simulink model "PendulumCart_sim"  (R2015a)
settings: Solver=ode45  StartTime=0.0  StopTime=30.0  RelTol=1e-3
InitFcn:
  | Ts = 0.02;
  | %SMC Parameters
  | lambda = 1; %surface
  | beta = 25;  %pull magnitude
  | U = 0.01;     %saturation
  | %system parameters
  | m = 0.2;
  | M = 0.5;
  | g = 9.8;
  | L = 0.3;
  | %system parameter estimates
  | m_hat = m;
  | M_hat = M;
  | g_hat = g;
  | L_hat = L;
libraries: simulink x1
settings Model: Creator=Logan  LastModifiedBy=Logan

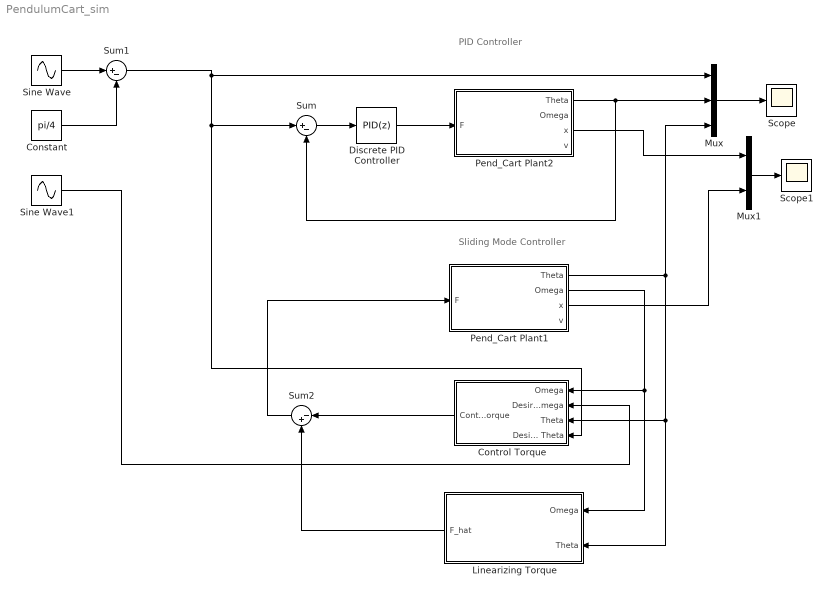
== system PendulumCart_sim ==
  note: PID Controller
  note: Sliding Mode Controller
  Constant : Constant  Value=pi/4
  Control Torque : Subsystem
  Discrete PID Controller : simulink/Continuous/PID Controller  Controller=PID  TimeDomain=Discrete-time  SampleTime=0.01  IntegratorMethod=Forward Euler  FilterMethod=Forward Euler  Form=Parallel  UseFilter=off  ControllerParametersSource=internal  P=100  I=1  D=20  N=250  InitialConditionSource=internal  InitialConditionForIntegrator=0  InitialConditionForFilter=0  ExternalReset=none  LimitOutput=off  UpperSaturationLimit=inf  LowerSaturationLimit=-inf  LinearizeAsGain=off  AntiWindupMode=none  Kb=1  TrackingMode=off  Kt=1  PParamMin=[]  PParamMax=[]  IParamMin=[]  IParamMax=[]  DParamMin=[]  DParamMax=[]  NParamMin=[]  NParamMax=[]  KbParamMin=[]  KbParamMax=[]  KtParamMin=[]  KtParamMax=[]  POutMin=[]  POutMax=[]  IOutMin=[]  IOutMax=[]  DOutMin=[]  DOutMax=[]  NOutMin=[]  NOutMax=[]  KbOutMin=[]  KbOutMax=[]  KtOutMin=[]  KtOutMax=[]  IntegratorOutMin=[]  IntegratorOutMax=[]  FilterOutMin=[]  FilterOutMax=[]  SumOutMin=[]  SumOutMax=[]  SumI1OutMin=[]  SumI1OutMax=[]  SumI2OutMin=[]  SumI2OutMax=[]  SumI3OutMin=[]  SumI3OutMax=[]  SumDOutMin=[]  SumDOutMax=[]  SaturationOutMin=[]  SaturationOutMax=[]  IntegratorContinuousStateAttributes=''  IntegratorStateMustResolveToSignalObject=off  IntegratorRTWStateStorageClass=Auto  FilterContinuousStateAttributes=''  FilterStateMustResolveToSignalObject=off  FilterRTWStateStorageClass=Auto  DifferentiatorICPrevScaledInput=0  DifferentiatorOutMin=[]  DifferentiatorOutMax=[]
  Linearizing Torque : Subsystem
  Mux : Mux  Inputs=3
  Mux1 : Mux  Inputs=2
  Pend_Cart Plant1 : Subsystem  VariantControl=Variant1
  Pend_Cart Plant2 : Subsystem  VariantControl=Variant1
  Scope : Scope
      settings: TimeRange=10  YMin=-1.5  YMax=7
  Scope1 : Scope
      settings: TimeRange=10  YMin=-3500  YMax=750  SaveName=PositionData
  Sine Wave : Sin  Amplitude=pi/8  Frequency=1/2  SampleTime=0
  Sine Wave1 : Sin  Amplitude=pi/16  Frequency=1/2  Phase=pi/2  SampleTime=0
  Sum : Sum  Inputs=|+-
  Sum1 : Sum  Inputs=|+-
  Sum2 : Sum  Inputs=|-+
  wires:
  Sum/1 -> Discrete PID Controller/1
  Mux/1 -> Scope/1
  Pend_Cart Plant1/1(Theta) -> Linearizing Torque/2(Theta), Control Torque/3(Theta), Mux/3
  Pend_Cart Plant1/2(Omega) -> Linearizing Torque/1(Omega), Control Torque/1(Omega)
  Linearizing Torque/1(F_hat) -> Sum2/2
  Sum2/1 -> Pend_Cart Plant1/1(F)
  Control Torque/1(Control Torque) -> Sum2/1
  Pend_Cart Plant2/1(Theta) -> Sum/2, Mux/2
  Discrete PID Controller/1 -> Pend_Cart Plant2/1(F)
  Sine Wave1/1 -> Control Torque/2(Desired Omega)
  Mux1/1 -> Scope1/1
  Pend_Cart Plant2/3(x) -> Mux1/1
  Pend_Cart Plant1/3(x) -> Mux1/2
  Sum1/1 -> Mux/1, Control Torque/4(Desired Theta), Sum/1
  Sine Wave/1 -> Sum1/1
  Constant/1 -> Sum1/2

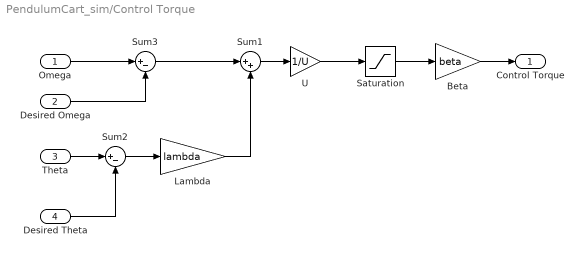
== system PendulumCart_sim/Control Torque ==
  Omega : Inport
  Desired Omega : Inport  Port=2
  Theta : Inport  Port=3
  Desired Theta : Inport  Port=4
  Beta : Gain  Gain=beta
  Lambda : Gain  Gain=lambda
  Saturation : Saturate  UpperLimit=1  LowerLimit=-1
  Sum1 : Sum  Inputs=|++
  Sum2 : Sum  Inputs=|+-
  Sum3 : Sum  Inputs=|+-
  U : Gain  Gain=1/U
  Control Torque : Outport
  wires:
  Lambda/1 -> Sum1/2
  Saturation/1 -> Beta/1
  Beta/1 -> Control Torque/1
  Sum2/1 -> Lambda/1
  U/1 -> Saturation/1
  Sum1/1 -> U/1
  Theta/1 -> Sum2/1
  Desired Theta/1 -> Sum2/2
  Omega/1 -> Sum3/1
  Sum3/1 -> Sum1/1
  Desired Omega/1 -> Sum3/2

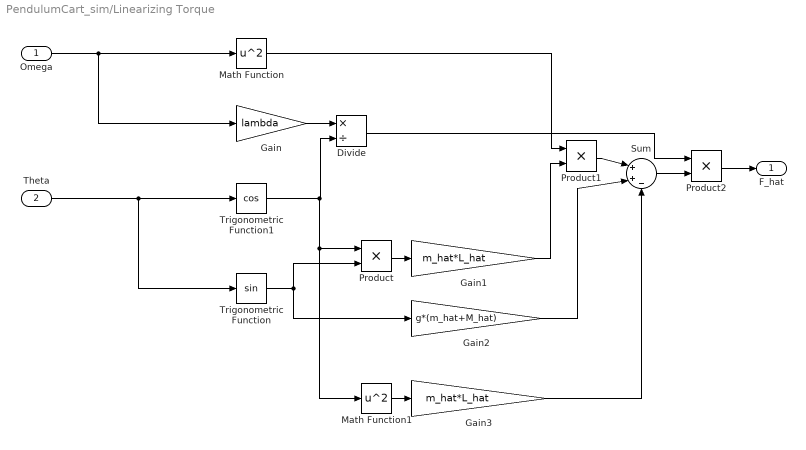
== system PendulumCart_sim/Linearizing Torque ==
  Omega : Inport
  Theta : Inport  Port=2
  Divide : Product  Inputs=*/
  Gain : Gain  Gain=lambda
  Gain1 : Gain  Gain=m_hat*L_hat
  Gain2 : Gain  Gain=g*(m_hat+M_hat)
  Gain3 : Gain  Gain=m_hat*L_hat
  Math Function : Math  Operator=square  SaturateOnIntegerOverflow=on
  Math Function1 : Math  Operator=square  SaturateOnIntegerOverflow=on
  Product : Product
  Product1 : Product
  Product2 : Product
  Sum : Sum  Inputs=|++-
  Trigonometric Function : Trigonometry
  Trigonometric Function1 : Trigonometry  Operator=cos
  F_hat : Outport
  wires:
  Theta/1 -> Trigonometric Function1/1, Trigonometric Function/1
  Omega/1 -> Gain/1, Math Function/1
  Gain/1 -> Divide/1
  Trigonometric Function1/1 -> Math Function1/1, Product/1, Divide/2
  Trigonometric Function/1 -> Product/2, Gain2/1
  Product/1 -> Gain1/1
  Gain1/1 -> Product1/2
  Product1/1 -> Sum/1
  Gain2/1 -> Sum/2
  Math Function1/1 -> Gain3/1
  Gain3/1 -> Sum/3
  Sum/1 -> Product2/2
  Divide/1 -> Product2/1
  Math Function/1 -> Product1/1
  Product2/1 -> F_hat/1

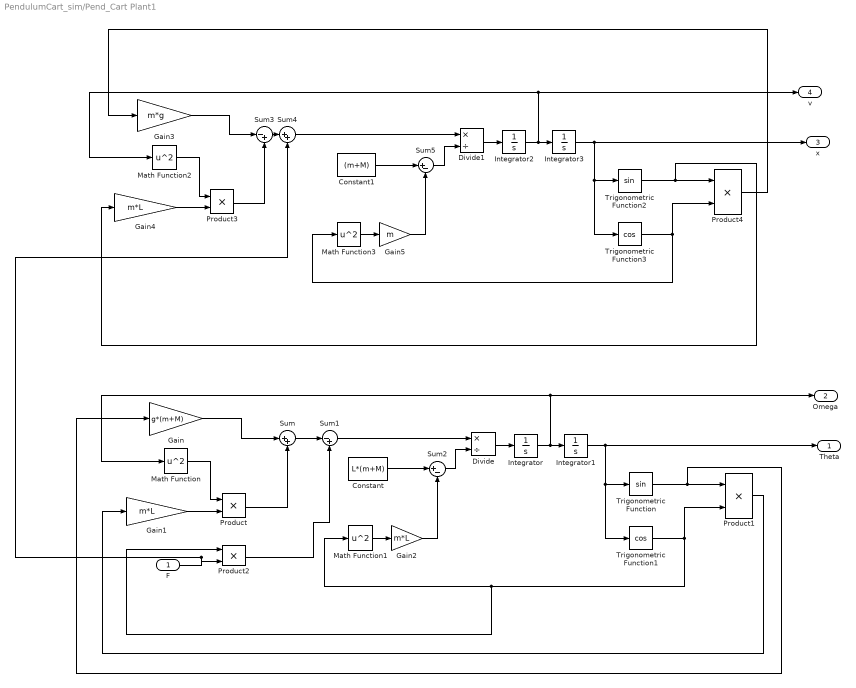
== system PendulumCart_sim/Pend_Cart Plant1 ==
  F : Inport
  Constant : Constant  Value=L*(m+M)
  Constant1 : Constant  Value=(m+M)
  Divide : Product  Inputs=*/
  Divide1 : Product  Inputs=*/
  Gain : Gain  Gain=g*(m+M)
  Gain1 : Gain  Gain=m*L
  Gain2 : Gain  Gain=m*L
  Gain3 : Gain  Gain=m*g
  Gain4 : Gain  Gain=m*L
  Gain5 : Gain  Gain=m
  Integrator : Integrator  InitialCondition=1
  Integrator1 : Integrator
  Integrator2 : Integrator  InitialCondition=1
  Integrator3 : Integrator
  Math Function{,1..3} (4 alike) : Math  Operator=square  SaturateOnIntegerOverflow=on
  Product{,1..4} (5 alike) : Product
  Sum : Sum  Inputs=|++
  Sum1 : Sum  Inputs=|-+
  Sum2 : Sum  Inputs=|+-
  Sum3 : Sum  Inputs=|-+
  Sum4 : Sum  Inputs=|++
  Sum5 : Sum  Inputs=|+-
  Trigonometric Function : Trigonometry
  Trigonometric Function1 : Trigonometry  Operator=cos
  Trigonometric Function2 : Trigonometry
  Trigonometric Function3 : Trigonometry  Operator=cos
  Theta : Outport
  Omega : Outport  Port=2
  x : Outport  Port=3
  v : Outport  Port=4
  wires:
  Product/1 -> Sum/2
  Gain/1 -> Sum/1
  Product2/1 -> Sum1/2
  Integrator1/1 -> Trigonometric Function1/1, Trigonometric Function/1, Theta/1
  Integrator/1 -> Integrator1/1, Omega/1, Math Function/1
  Divide/1 -> Integrator/1
  Sum2/1 -> Divide/2
  Sum1/1 -> Divide/1
  Constant/1 -> Sum2/1
  Gain2/1 -> Sum2/2
  Math Function1/1 -> Gain2/1
  Math Function/1 -> Product/1
  Gain1/1 -> Product/2
  Trigonometric Function/1 -> Gain/1, Product1/1
  Product1/1 -> Gain1/1
  Trigonometric Function1/1 -> Product2/1, Math Function1/1, Product1/2
  Sum/1 -> Sum1/1
  Product3/1 -> Sum3/2
  Gain3/1 -> Sum3/1
  F/1 -> Sum4/2, Product2/2
  Integrator3/1 -> x/1, Trigonometric Function3/1, Trigonometric Function2/1
  Integrator2/1 -> Integrator3/1, v/1, Math Function2/1
  Divide1/1 -> Integrator2/1
  Sum5/1 -> Divide1/2
  Sum4/1 -> Divide1/1
  Constant1/1 -> Sum5/1
  Gain5/1 -> Sum5/2
  Math Function3/1 -> Gain5/1
  Math Function2/1 -> Product3/1
  Gain4/1 -> Product3/2
  Trigonometric Function2/1 -> Gain4/1, Product4/1
  Trigonometric Function3/1 -> Math Function3/1, Product4/2
  Sum3/1 -> Sum4/1
  Product4/1 -> Gain3/1

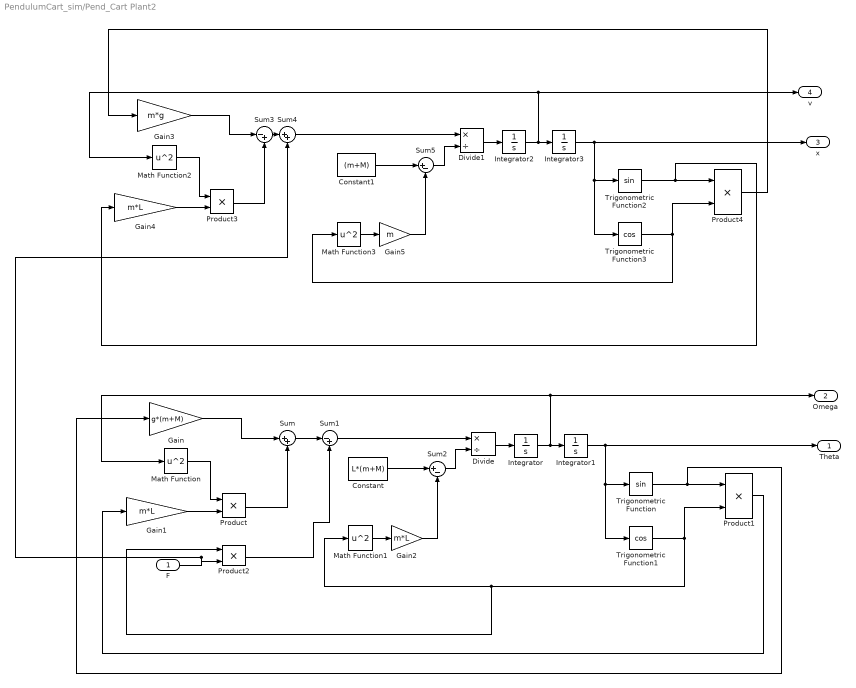
== system PendulumCart_sim/Pend_Cart Plant2 ==
  F : Inport
  Constant : Constant  Value=L*(m+M)
  Constant1 : Constant  Value=(m+M)
  Divide : Product  Inputs=*/
  Divide1 : Product  Inputs=*/
  Gain : Gain  Gain=g*(m+M)
  Gain1 : Gain  Gain=m*L
  Gain2 : Gain  Gain=m*L
  Gain3 : Gain  Gain=m*g
  Gain4 : Gain  Gain=m*L
  Gain5 : Gain  Gain=m
  Integrator : Integrator  InitialCondition=1
  Integrator1 : Integrator
  Integrator2 : Integrator  InitialCondition=1
  Integrator3 : Integrator
  Math Function{,1..3} (4 alike) : Math  Operator=square  SaturateOnIntegerOverflow=on
  Product{,1..4} (5 alike) : Product
  Sum : Sum  Inputs=|++
  Sum1 : Sum  Inputs=|-+
  Sum2 : Sum  Inputs=|+-
  Sum3 : Sum  Inputs=|-+
  Sum4 : Sum  Inputs=|++
  Sum5 : Sum  Inputs=|+-
  Trigonometric Function : Trigonometry
  Trigonometric Function1 : Trigonometry  Operator=cos
  Trigonometric Function2 : Trigonometry
  Trigonometric Function3 : Trigonometry  Operator=cos
  Theta : Outport
  Omega : Outport  Port=2
  x : Outport  Port=3
  v : Outport  Port=4
  wires:
  Product/1 -> Sum/2
  Gain/1 -> Sum/1
  Product2/1 -> Sum1/2
  Integrator1/1 -> Trigonometric Function1/1, Trigonometric Function/1, Theta/1
  Integrator/1 -> Integrator1/1, Omega/1, Math Function/1
  Divide/1 -> Integrator/1
  Sum2/1 -> Divide/2
  Sum1/1 -> Divide/1
  Constant/1 -> Sum2/1
  Gain2/1 -> Sum2/2
  Math Function1/1 -> Gain2/1
  Math Function/1 -> Product/1
  Gain1/1 -> Product/2
  Trigonometric Function/1 -> Gain/1, Product1/1
  Product1/1 -> Gain1/1
  Trigonometric Function1/1 -> Product2/1, Math Function1/1, Product1/2
  Sum/1 -> Sum1/1
  Product3/1 -> Sum3/2
  Gain3/1 -> Sum3/1
  F/1 -> Sum4/2, Product2/2
  Integrator3/1 -> x/1, Trigonometric Function3/1, Trigonometric Function2/1
  Integrator2/1 -> Integrator3/1, v/1, Math Function2/1
  Divide1/1 -> Integrator2/1
  Sum5/1 -> Divide1/2
  Sum4/1 -> Divide1/1
  Constant1/1 -> Sum5/1
  Gain5/1 -> Sum5/2
  Math Function3/1 -> Gain5/1
  Math Function2/1 -> Product3/1
  Gain4/1 -> Product3/2
  Trigonometric Function2/1 -> Gain4/1, Product4/1
  Trigonometric Function3/1 -> Math Function3/1, Product4/2
  Sum3/1 -> Sum4/1
  Product4/1 -> Gain3/1
